simulink model "Esempio4_s"  (R2021b)
settings: Solver=VariableStepAuto  StartTime=0.0  StopTime=10.0  RelTol=1e-3
undefined symbols (not defined in the file): A, B, C, K, x0
settings Model: Creator=Steph  LastModifiedBy=Steph

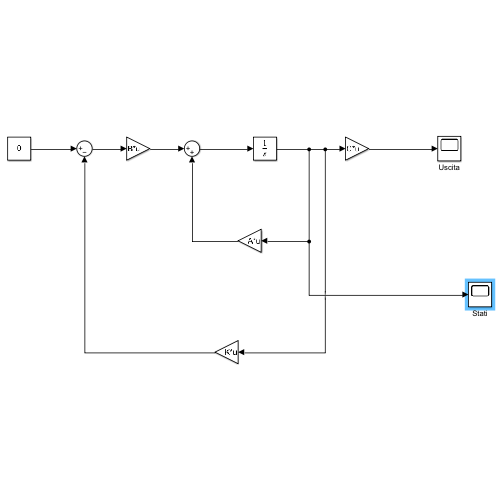
[thumbnail: Simulink's stored preview of the top-level diagram]
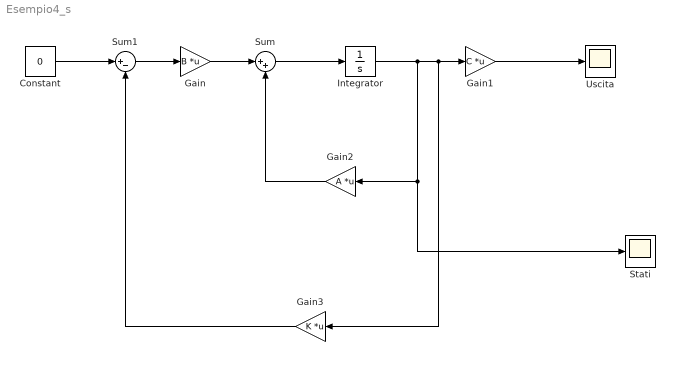
== system Esempio4_s ==
  Constant : Constant  Value=0
  Gain : Gain  Gain=B  Multiplication=Matrix(K*u)
  Gain1 : Gain  Gain=C  Multiplication=Matrix(K*u)
  Gain2 : Gain  Gain=A  Multiplication=Matrix(K*u)
  Gain3 : Gain  Gain=K  Multiplication=Matrix(K*u)
  Integrator : Integrator  InitialCondition=x0
  Stati : Scope
  Sum : Sum  Inputs=|++
  Sum1 : Sum  Inputs=|+-
  Uscita : Scope
  wires:
  Gain3/1 -> Sum1/2
  Integrator/1 -> Stati/1, Gain2/1, Gain3/1, Gain1/1
  Gain1/1 -> Uscita/1
  Sum/1 -> Integrator/1
  Gain/1 -> Sum/1
  Gain2/1 -> Sum/2
  Sum1/1 -> Gain/1
  Constant/1 -> Sum1/1
